simulink subsystem "subrPID"  (R2024a)
settings: Solver=VariableStepAuto  StartTime=0.0  StopTime=10.0  RelTol=1e-3
model mask{Kp=0, Ki=0, Kd=0, Ki_Sat=inf, TSTEP=-1}
  mask prompts: Kp "Proportional Gain"; Ki "Integral Gain"; Kd "Derivative Gain"; Ki_Sat "Integrator Saturation"; TSTEP "Time Step"
settings Model: Creator=anant  LastModifiedBy=anant

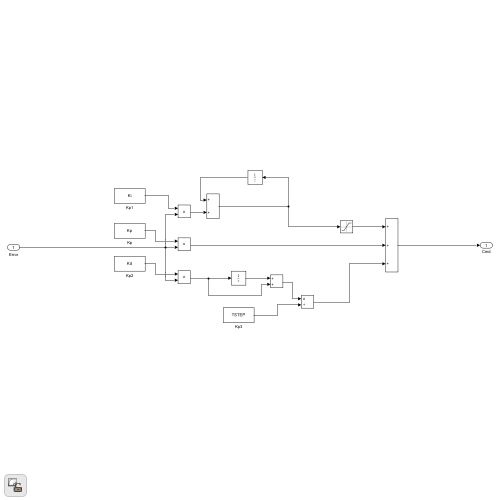
[thumbnail: Simulink's stored preview of the top-level diagram]
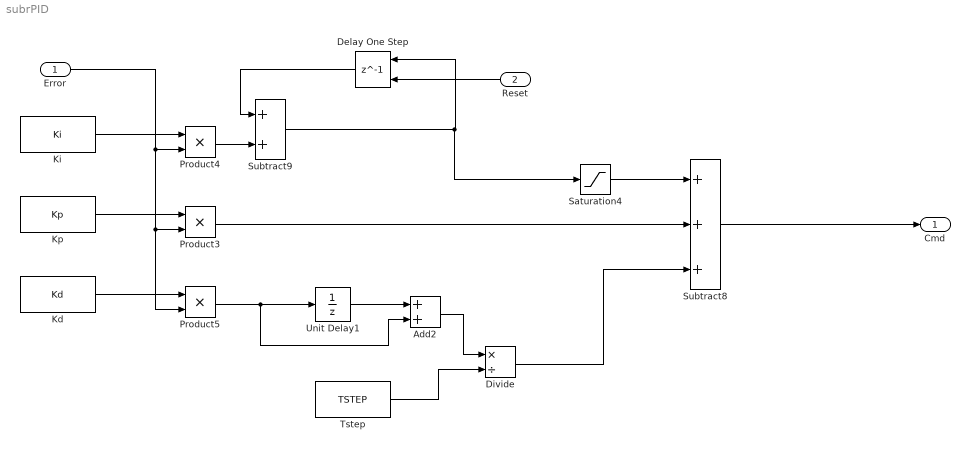
== system subrPID ==
  Error : Inport
  Reset : Inport  Port=2
  Add2 : Sum
  Delay One Step : Delay  DelayLength=1  ExternalReset=Rising  SampleTime=TSTEP
      settings: InputPortMap=u0,r5
  Divide : Product  Inputs=*/
  Kd : Constant  Value=Kd
  Ki : Constant  Value=Ki
  Kp : Constant  Value=Kp
  Product3 : Product
  Product4 : Product
  Product5 : Product
  Saturation4 : Saturate  UpperLimit=Ki_Sat  LowerLimit=-Ki_Sat
  Subtract8 : Sum  Inputs=+++
  Subtract9 : Sum
  Tstep : Constant  Value=TSTEP
  Unit Delay1 : UnitDelay  SampleTime=TSTEP  HasFrameUpgradeWarning=on
  Cmd : Outport
  wires:
  Kp/1 -> Product3/1
  Tstep/1 -> Divide/2
  Error/1 -> Product4/2, Product3/2, Product5/2
  Kd/1 -> Product5/1
  Delay One Step/1 -> Subtract9/1
  Product5/1 -> Unit Delay1/1, Add2/2
  Subtract8/1 -> Cmd/1
  Unit Delay1/1 -> Add2/1
  Product4/1 -> Subtract9/2
  Divide/1 -> Subtract8/3
  Product3/1 -> Subtract8/2
  Add2/1 -> Divide/1
  Saturation4/1 -> Subtract8/1
  Ki/1 -> Product4/1
  Reset/1 -> Delay One Step/2
  Subtract9/1 -> Delay One Step/1, Saturation4/1
